simulink model "chap6_7sim"  (Simulink 5.0)
settings: Solver=ode45  StartTime=0.0  StopTime=16  FixedStep=0.001  RelTol=1e-3
settings Model: LastModifiedBy=Administrator  ExtModeTrigMode=oneshot  ExtModeArmWhenConnect=off  LimitDataPoints=off  BooleanDataType=off

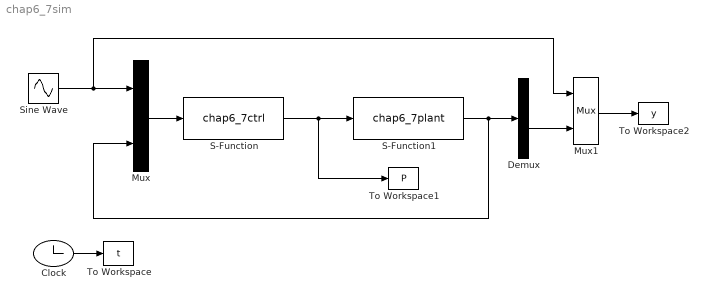
== system chap6_7sim ==
  Clock : Clock
  Demux : Demux
  Mux : Mux  Inputs=2
  Mux1 : Mux  Inputs=2
  S-Function : S-Function  FunctionName=chap6_7ctrl
  S-Function1 : S-Function  FunctionName=chap6_7plant
  Sine Wave : Sin  SampleTime=0
  To Workspace : ToWorkspace  VariableName=t  SampleTime=-1  SaveFormat=Array
  To Workspace1 : ToWorkspace  VariableName=P  SampleTime=-1  SaveFormat=Array
  To Workspace2 : ToWorkspace  VariableName=y  SampleTime=-1  SaveFormat=Array
  wires:
  Sine Wave/1 -> Mux1/1, Mux/1
  Mux1/1 -> To Workspace2/1
  S-Function1/1 -> Mux/2, Demux/1
  Mux/1 -> S-Function/1
  Demux/3 -> Mux1/2
  Clock/1 -> To Workspace/1
  S-Function/1 -> S-Function1/1, To Workspace1/1
